simulink model "recoveryattempt_top_model"  (R2024b)
settings: Solver=VariableStepAuto  StartTime=0.0  StopTime=1000  FixedStep=0.001  RelTol=1e-6  EnableMultiTasking=on
undefined symbols (not defined in the file): ClassLabel, ClassValidity, controller, gray, imageEnums, images, pointsOfWay, vehicle, world, X, Y, Z
libraries: sm_lib x44, simulink x7, nesl_utility x7, slpidlib x2, deeplib x1, dspstat3 x1, robotmobilelib x1
(part 1 of 2)
settings Model: Creator=The MathWorks, Inc.  LastModifiedBy=carla
settings SolverCC: AlgebraicLoopSolver=TrustRegion  AutoInsertRateTranBlk=on
settings DataIOCC: LimitDataPoints=on  ReturnWorkspaceOutputs=off
settings OptimizationCC: LifeSpan=inf
settings DebuggingCC: AlgebraicLoopMsg=none  UnconnectedInputMsg=warning  UnconnectedOutputMsg=warning  UnconnectedLineMsg=warning  AllowSymbolicDim=off  SFUnexpectedBacktrackingDiag=warning  SFNoUnconditionalDefaultTransitionDiag=warning  SFExecutionAtInitializationDiag=none  ArithmeticOperatorsInVariantConditions=warning
settings ModelReferenceCC: EnableRefExpFcnMdlSchedulingChecks=on  PropagateSignalLabelsOutOfModel=off
settings SFSimCC: SimUseLocalCustomCode=off  CustomCodeUndefinedFunction=UseInterfaceOnly
settings RTWCC: RTWUseLocalCustomCode=off  GPUComputeCapability=3.5
settings CodeAppCC: StateflowObjectComments=on
settings GRTTargetCC: TargetLangStandard=C89/C90 (ANSI)
settings ConfigComp: CovMetricSettings=dw  CovSaveCumulativeToWorkspaceVar=on  CovSaveSingleToWorkspaceVar=on  CovExternalEMLEnable=off
settings ExplorerConfigSet: InternalSimMechanicsExplorerSettings="<ExplorerConfiguration><canonicalview>default</canonicalview><AnimationSetting><BasePlaybackSpeed>1.0</BasePlaybackSpeed><PlaybackSpeedFactor>4.0</PlaybackSpeedFactor></AnimationSetting><TilePanel><TileInfo><Tiles Columns=\"1\" Count=\"1\" Rows=\"1\"><Column Weight=\"1\"/><Row Weight=\"1\"/><Tile Height=\"1\" Width=\"1\" X=\"0\" Y=\"0\"/></Tiles></TileInfo><SceneInfo><SceneViewer><BGColor><R>0.60000002384185791</R><G>0.60000002384185791</G><B>0.60000002384185791</B></BGColor><Camera><DoPerspective>off</DoPerspective><Position><X>30.3692307922621794</X><Y>-2.86922998928845274</Y><Z>15.3692305721881048</Z></Position><Center><X>14.9999996252394148</X><Y>12.5000011777343119</Y><Z>-5.94834646427955249e-07</Z></Center><Up><X>-0.408248290463863073</X><Y>0.408248290463863073</Y><Z>0.816496580927726145</Z></Up><ViewLimDist>1</ViewLimDist><YLim>15.7961190654270691</YLim><XLim>27.3119994163513198</XLim></Camera></SceneViewer></SceneInfo></TilePanel><MechEditorPanel><Cameras/><GfxPanelCameraMap/><VideoCreator><PlaybackSpeedRatio>4.0</PlaybackSpeedRatio><FrameRate>30</FrameRate><VideoFormat>MPEG-4</VideoFormat><FrameSize>auto</FrameSize></VideoCreator></MechEditorPanel></ExplorerConfiguration>"

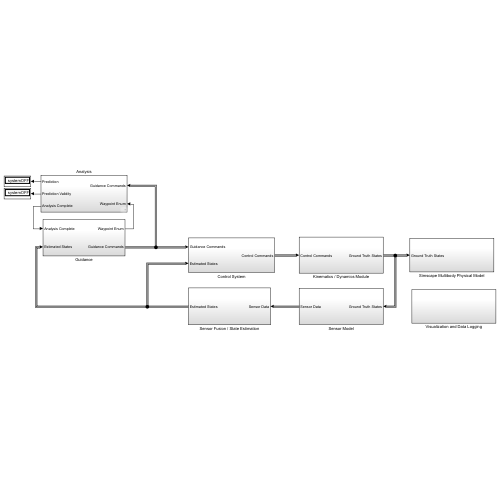
[thumbnail: Simulink's stored preview of the top-level diagram]
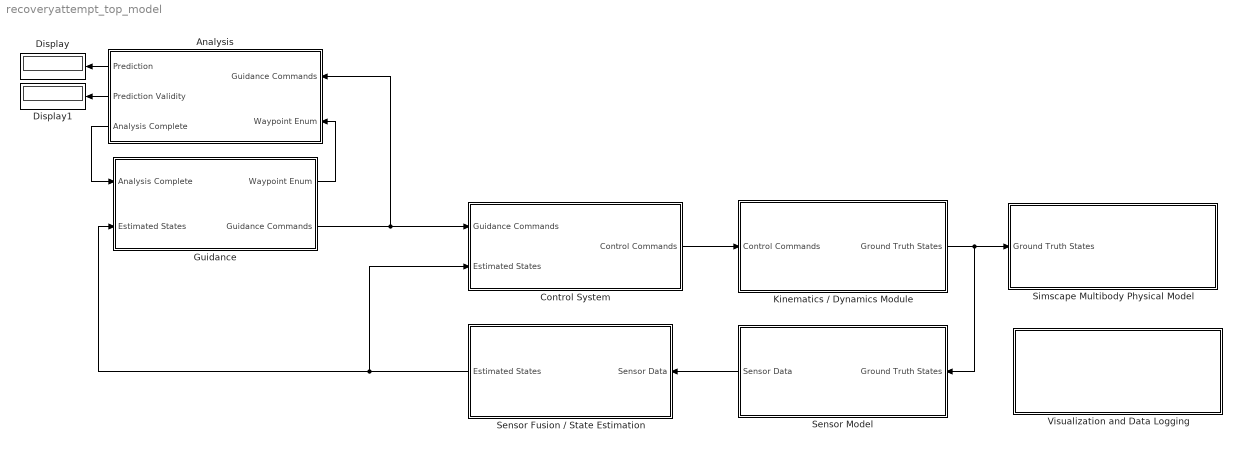
== system recoveryattempt_top_model ==
  Analysis : Subsystem
  Control System : Subsystem
  Display : Display
  Display1 : Display
  Guidance : Subsystem
  Kinematics / Dynamics Module : Subsystem
  Sensor Fusion / State Estimation : Subsystem
  Sensor Model : Subsystem
  Simscape Multibody Physical Model : Subsystem
  Visualization and Data Logging : Subsystem
  wires:
  Sensor Model/1(Sensor Data) -> Sensor Fusion / State Estimation/1(Sensor Data)
  Control System/1(Control Commands) -> Kinematics / Dynamics Module/1(Control Commands)
  Kinematics / Dynamics Module/1(Ground Truth States) -> Simscape Multibody Physical Model/1(Ground Truth States), Sensor Model/1(Ground Truth States)
  Sensor Fusion / State Estimation/1(Estimated States) -> Control System/2(Estimated States), Guidance/2(Estimated States)
  Analysis/1(Prediction) -> Display/1
  Guidance/2(Guidance Commands) -> Analysis/1(Guidance Commands), Control System/1(Guidance Commands)
  Analysis/3(Analysis Complete) -> Guidance/1(Analysis Complete)
  Guidance/1(Waypoint Enum) -> Analysis/2(Waypoint Enum)
  Analysis/2(Prediction Validity) -> Display1/1

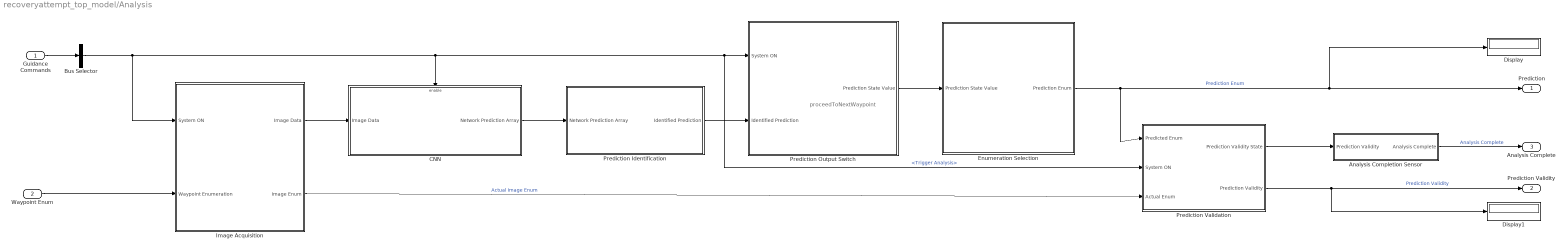
== system recoveryattempt_top_model/Analysis ==
  note: proceedToNextWaypoint
  Guidance Commands : Inport
  Waypoint Enum : Inport  Port=2
  Analysis Completion Sensor : Subsystem
  Bus Selector : BusSelector  OutputSignals=Process Commands.Trigger Analysis
  CNN : Subsystem
  Display : Display
  Display1 : Display
  Enumeration Selection : Subsystem
  Image Acquisition : Subsystem
  Prediction Identification : Subsystem
  Prediction Output Switch : Subsystem
  Prediction Validation : Subsystem
  Prediction : Outport
  Prediction Validity : Outport  Port=2
  Analysis Complete : Outport  Port=3
  wires:
  Waypoint Enum/1 -> Image Acquisition/2(Waypoint Enumeration)
  Image Acquisition/1(Image Data) -> CNN/1(Image Data)
  Bus Selector/1 -> Image Acquisition/1(System ON), CNN/Enable, Prediction Validation/2(System ON), Prediction Output Switch/1(System ON)  "<Trigger Analysis>"
  Guidance Commands/1 -> Bus Selector/1
  Prediction Identification/1(Identified Prediction) -> Prediction Output Switch/2(Identified Prediction)
  CNN/1(Network Prediction Array) -> Prediction Identification/1(Network Prediction Array)
  Enumeration Selection/1(Prediction Enum) -> Prediction Validation/1(Predicted Enum), Prediction/1, Display/1  "Prediction Enum"
  Prediction Output Switch/1(Prediction State Value) -> Enumeration Selection/1(Prediction State Value)
  Image Acquisition/2(Image Enum) -> Prediction Validation/3(Actual Enum)  "Actual Image Enum"
  Prediction Validation/2(Prediction Validity) -> Display1/1, Prediction Validity/1  "Prediction Validity"
  Analysis Completion Sensor/1(Analysis Complete) -> Analysis Complete/1  "Analysis Complete"
  Prediction Validation/1(Prediction Validity State) -> Analysis Completion Sensor/1(Prediction Validity)

== system recoveryattempt_top_model/Control System ==
  Guidance Commands : Inport
  Estimated States : Inport  Port=2
  Bus Selector : BusSelector  OutputSignals=Target Waypoints,Event Flags.Target Waypoint Reached
  Bus Selector1 : BusSelector  OutputSignals=True Position States
  Control Logic : Subsystem
  Control Commands : Outport
  wires:
  Estimated States/1 -> Bus Selector1/1
  Bus Selector/1 -> Control Logic/1(Target Waypoints)  "<Target Waypoints>"
  Guidance Commands/1 -> Bus Selector/1
  Control Logic/1(Control Commands) -> Control Commands/1
  Bus Selector1/1 -> Control Logic/3(Estimated Position)  "<True Position States>"
  Bus Selector/2 -> Control Logic/2(Target Waypoint Reached)  "<Target Waypoint Reached>"

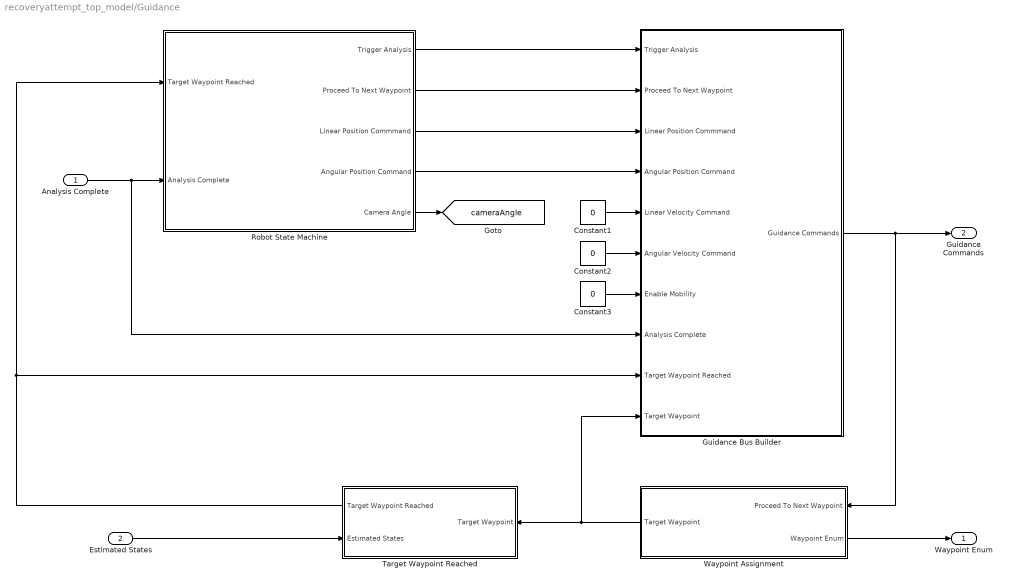
== system recoveryattempt_top_model/Guidance ==
  Analysis Complete : Inport
  Estimated States : Inport  Port=2
  Constant1 : Constant  Value=0
  Constant2 : Constant  Value=0
  Constant3 : Constant  Value=0
  Guidance Bus Builder : Subsystem
  Robot State Machine : Subsystem
  Target Waypoint Reached : Subsystem
      settings: PortSchema="{\"entries\":[{\"content\":{\"sides\":[{\"content\":{\"connectorIds\":[\"Out1\",\"In1\"]},\"type\":\"ConnectorPlacement.EquallySpacedRectSide\",\"uuid\":\"d7010085-5ef5-4f49-a809-03aff96e46a3\"},{\"content\":{\"connectorIds\":[\"In2\"],\"side\":\"RIGHT\"},\"type\":\"ConnectorPlacement.EquallySpacedRectSide\",\"uuid\":\"23b66111-6f3c-45e8-b3ba-0f5bee8484ca\"},{\"content\":{\"side\":\"TOP\"},\"type\":\"ConnectorPlacement.EquallySpacedRectSide\",\"uuid\":\"a521ae1c-357f-4992-b141-24939590eede\"}]},\"type\":\"ConnectorPlacement.EquallySpacedConnector\",\"uuid\":\"a962b4e6-4c12-48b9-996e-c7d697d970f0\"}],\"packageUris\":[\"http://schema.mathworks.com/mf0/Connector/R2020b\"],\"version\":\"1.0\"}"
  "Waypoint Assignment " : Subsystem
      settings: PortSchema="{\"entries\":[{\"content\":{\"sides\":[{\"content\":{\"connectorIds\":[\"In1\",\"Out2\"]},\"type\":\"ConnectorPlacement.EquallySpacedRectSide\",\"uuid\":\"23aedb4f-9300-4426-912f-0e2d5fd3b29f\"},{\"content\":{\"connectorIds\":[\"Out1\"],\"side\":\"RIGHT\"},\"type\":\"ConnectorPlacement.EquallySpacedRectSide\",\"uuid\":\"0851e076-2bde-4b70-9977-919ee7e7eb4f\"},{\"content\":{\"side\":\"TOP\"},\"type\":\"ConnectorPlacement.EquallySpacedRectSide\",\"uuid\":\"d0edf62d-75f3-4cec-8020-5fb7633b53e3\"}]},\"type\":\"ConnectorPlacement.EquallySpacedConnector\",\"uuid\":\"92e9c851-2c74-435e-8a22-f69b21df6f3e\"}],\"packageUris\":[\"http://schema.mathworks.com/mf0/Connector/R2020b\"],\"version\":\"1.0\"}"
  Waypoint Enum : Outport
  Guidance Commands : Outport  Port=2
  tag scope: cameraAngle=global
  wires:
  Robot State Machine/1(Trigger Analysis) -> Guidance Bus Builder/1(Trigger Analysis)
  Constant1/1 -> Guidance Bus Builder/5(Linear Velocity Command)
  Constant2/1 -> Guidance Bus Builder/6(Angular Velocity Command)
  Robot State Machine/4(Angular Position Command) -> Guidance Bus Builder/4(Angular Position Command)
  Robot State Machine/3(Linear Position Commmand) -> Guidance Bus Builder/3(Linear Position Commmand)
  Constant3/1 -> Guidance Bus Builder/7(Enable Mobility)
  Analysis Complete/1 -> Robot State Machine/2(Analysis Complete), Guidance Bus Builder/8(Analysis Complete)
  Robot State Machine/2(Proceed To Next Waypoint) -> Guidance Bus Builder/2(Proceed To Next Waypoint)
  Target Waypoint Reached/1(Target Waypoint Reached) -> Guidance Bus Builder/9(Target Waypoint Reached), Robot State Machine/1(Target Waypoint Reached)
  Guidance Bus Builder/1(Guidance Commands) -> Guidance Commands/1, "Waypoint Assignment "/1(Proceed To Next Waypoint)
  "Waypoint Assignment "/1(Target Waypoint) -> Guidance Bus Builder/10(Target Waypoint), Target Waypoint Reached/2(Target Waypoint)
  Estimated States/1 -> Target Waypoint Reached/1(Estimated States)
  Robot State Machine/5(Camera Angle) -> [cameraAngle]
  "Waypoint Assignment "/2(Waypoint Enum) -> Waypoint Enum/1

== system recoveryattempt_top_model/Kinematics // Dynamics Module ==
  Control Commands : Inport
  Bus Creator : BusCreator  Inputs=3
  Bus Creator1 : BusCreator  Inputs=3
  Bus Creator2 : BusCreator  Inputs=2
  Bus Selector : BusSelector  OutputSignals=Linear Velocity Command,Angular Velocity Command
  Demux1 : Demux  Outputs=3
  Demux2 : Demux  Outputs=3
  Differential Drive Kinematic Model : robotmobilelib/Differential Drive Kinematic Model  VehicleInputs=Vehicle Speed & Heading Angular Velocity  WheelRadius=vehicle.wheel.radius  WheelSpeedRange=[-inf inf]  TrackWidth=vehicle.wheel.width  InitialState=init.vehicle.state  SimulateUsing=Interpreted execution
  Ground Truth States : Outport
  wires:
  Bus Selector/1 -> Differential Drive Kinematic Model/1  "<Linear Velocity Command>"
  Bus Selector/2 -> Differential Drive Kinematic Model/2  "<Angular Velocity Command>"
  Control Commands/1 -> Bus Selector/1
  Differential Drive Kinematic Model/1 -> Demux1/1
  Demux1/2 -> Bus Creator/2  "True Position Y"
  Demux1/1 -> Bus Creator/1  "True Position X"
  Demux1/3 -> Bus Creator/3  "True Orientation"
  Differential Drive Kinematic Model/2 -> Demux2/1
  Demux2/1 -> Bus Creator1/1  "True Linear Velocity X"
  Demux2/3 -> Bus Creator1/3  "True Angular Velocity"
  Demux2/2 -> Bus Creator1/2  "True Linear Velocity Y"
  Bus Creator/1 -> Bus Creator2/1  "True Position States"
  Bus Creator1/1 -> Bus Creator2/2  "True Velocity States"
  Bus Creator2/1 -> Ground Truth States/1  "Ground Truth States"

== system recoveryattempt_top_model/Sensor Fusion // State Estimation ==
  Sensor Data : Inport
  Bus Creator : BusCreator  Inputs=2
  Bus Selector : BusSelector  OutputSignals=True Position States,True Velocity States
  Sensor Fusion : Subsystem
  Estimated States : Outport
  wires:
  Sensor Data/1 -> Bus Selector/1  "Sensor Data"
  Bus Creator/1 -> Estimated States/1  "Estimated States"
  Bus Selector/1 -> Sensor Fusion/1(In1)  "<True Position States>"
  Bus Selector/2 -> Sensor Fusion/2(In2)  "<True Velocity States>"
  Sensor Fusion/1(Out1) -> Bus Creator/1
  Sensor Fusion/2(Out2) -> Bus Creator/2

== system recoveryattempt_top_model/Sensor Model ==
  Ground Truth States : Inport
  Sensors : Subsystem
  Switch : simulink/Signal Routing/Manual Variant Source  NumChoices=2  LabelModeActiveChoice=V_1
  True Feedthrough : Subsystem
  Sensor Data : Outport
  wires:
  Switch/1 -> Sensor Data/1
  Ground Truth States/1 -> True Feedthrough/1(Ground Truth States), Sensors/1(Ground Truth States)
  Sensors/1(Simulated Raw Sensor Data) -> Switch/1  "Sensor Data"
  True Feedthrough/1(True Feedthrough Sensor Data) -> Switch/2  "Sensor Data"

== system recoveryattempt_top_model/Simscape Multibody Physical Model ==
  Ground Truth States : Inport
  Bus Creator : BusCreator  Inputs=1
  Bus Selector : BusSelector  OutputSignals=True Position States
  Bus Selector1 : BusSelector  OutputSignals=Camera Angle
  Simscape Model : Subsystem
  wires:
  Ground Truth States/1 -> Bus Selector/1
  Bus Selector/1 -> Simscape Model/1(True Position States)  "<True Position States>"
  Bus Selector1/1 -> Simscape Model/2(Peripheral Commands)  "<Camera Angle>"
  [cameraAngle] -> Bus Creator/1  "Camera Angle"
  Bus Creator/1 -> Bus Selector1/1  "Peripheral Commands"

== system recoveryattempt_top_model/Visualization and Data Logging ==

== system recoveryattempt_top_model/Analysis/Analysis Completion Sensor ==
  Prediction Validity : Inport
  Compare To Constant2 : simulink/Logic and Bit Operations/Compare To Constant  relop=<  const=2  OutDataTypeStr=boolean
  Display : Display
  Display1 : Display
  Analysis Complete : Outport
  wires:
  Prediction Validity/1 -> Display/1, Compare To Constant2/1
  Compare To Constant2/1 -> Analysis Complete/1, Display1/1

== system recoveryattempt_top_model/Analysis/CNN ==
  Image Data : Inport
  <Trigger Analysis> : EnablePort
  Predict : deeplib/Predict  Network=Network from MAT-file  NetworkFunction=squeezenet  NetworkFilePath=cleanTomatoNet.mat  MiniBatchSize=128  InputDataFormats={'',''}  Predictions=on  Activations={}  ForceInterpretedSim=off  EnableDLNetwork=on  LastKnownNetworkFilePath=''  LastKnownNetworkTimeStamp=''
  Network Prediction Array : Outport
  wires:
  Image Data/1 -> Predict/1
  Predict/1 -> Network Prediction Array/1

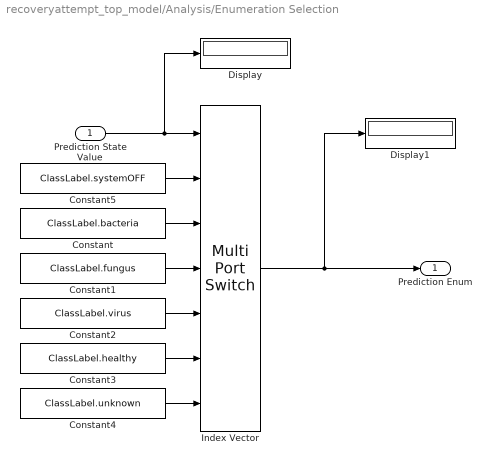
== system recoveryattempt_top_model/Analysis/Enumeration Selection ==
  Prediction State Value : Inport
  Constant : Constant  Value=ClassLabel.bacteria
  Constant1 : Constant  Value=ClassLabel.fungus
  Constant2 : Constant  Value=ClassLabel.virus
  Constant3 : Constant  Value=ClassLabel.healthy
  Constant4 : Constant  Value=ClassLabel.unknown
  Constant5 : Constant  Value=ClassLabel.systemOFF
  Display : Display
  Display1 : Display
  Index Vector : MultiPortSwitch  DataPortOrder=Zero-based contiguous  Inputs=6  zeroidx=on  SaturateOnIntegerOverflow=off  InputSameDT=off
  Prediction Enum : Outport
  wires:
  Index Vector/1 -> Prediction Enum/1, Display1/1
  Constant5/1 -> Index Vector/2
  Constant3/1 -> Index Vector/6
  Constant/1 -> Index Vector/3
  Constant4/1 -> Index Vector/7
  Constant1/1 -> Index Vector/4
  Constant2/1 -> Index Vector/5
  Prediction State Value/1 -> Index Vector/1, Display/1

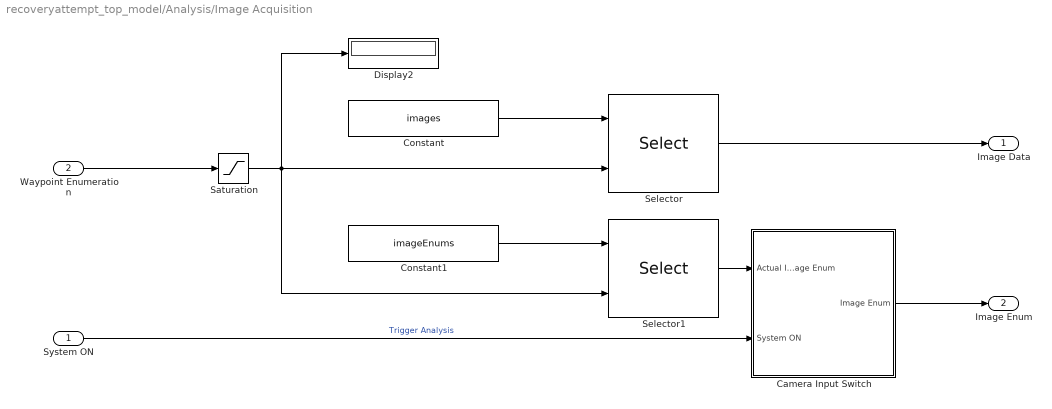
== system recoveryattempt_top_model/Analysis/Image Acquisition ==
  System ON : Inport
  Waypoint Enumeration : Inport  Port=2
  Camera Input Switch : Subsystem
  Constant : Constant  Value=images
  Constant1 : Constant  Value=imageEnums
  Display2 : Display
  Saturation : Saturate  UpperLimit=length(pointsOfWay)-1  LowerLimit=1
  Selector : Selector  NumberOfDimensions=4  InputPortWidth=3  IndexOptions=Select all,Select all,Select all,Index vector (port)  Indices=[1 3],1,1,1  OutputSizes=1,1,1,1
  Selector1 : Selector  InputPortWidth=36  IndexOptions=Index vector (port)  Indices=[1 3]  OutputSizes=1
  Image Data : Outport
  Image Enum : Outport  Port=2
  wires:
  Selector/1 -> Image Data/1
  Constant/1 -> Selector/1
  Constant1/1 -> Selector1/1
  Camera Input Switch/1(Image Enum) -> Image Enum/1
  Selector1/1 -> Camera Input Switch/1(Actual Image Enum)
  System ON/1 -> Camera Input Switch/2(System ON)  "Trigger Analysis"
  Waypoint Enumeration/1 -> Saturation/1
  Saturation/1 -> Selector1/2, Display2/1, Selector/2

== system recoveryattempt_top_model/Analysis/Prediction Identification ==
  Network Prediction Array : Inport
  Display : Display
  Display1 : Display
  Maximum : dspstat3/Maximum  operation=maximum  fcn=Index  indexBase=One  operateOver=Each row  Dimension=1  InputProcessing=Columns as channels (frame based)  reset=None  roiEnable=off  roiType=Rectangles  roiPortion=Entire ROI  roiOutput=Individual statistics for each ROI  roiFlag=off  roundingMode=Floor  overflowMode=off  accumDataTypeStr=Inherit: Same as product output  accumLastDataTypeStr=Inherit: Same as product output
  Identified Prediction : Outport
  wires:
  Network Prediction Array/1 -> Maximum/1, Display/1
  Maximum/1 -> Identified Prediction/1, Display1/1

== system recoveryattempt_top_model/Analysis/Prediction Output Switch ==
  System ON : Inport
  Identified Prediction : Inport  Port=2
  CNN OFF Value : Constant  Value=0
  Display : Display
  Display1 : Display
  Switch : Switch  Criteria=u2 > Threshold  SaturateOnIntegerOverflow=off  InputSameDT=off
  Prediction State Value : Outport
  wires:
  CNN OFF Value/1 -> Switch/3
  Switch/1 -> Prediction State Value/1, Display1/1
  Identified Prediction/1 -> Switch/1, Display/1
  System ON/1 -> Switch/2

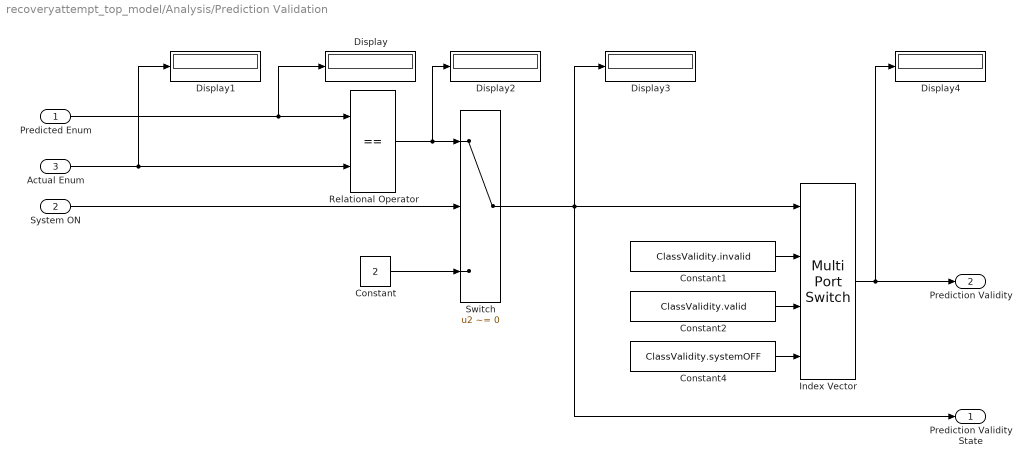
== system recoveryattempt_top_model/Analysis/Prediction Validation ==
  Predicted Enum : Inport
  System ON : Inport  Port=2
  Actual Enum : Inport  Port=3
  Constant : Constant  Value=2
  Constant1 : Constant  Value=ClassValidity.invalid
  Constant2 : Constant  Value=ClassValidity.valid
  Constant4 : Constant  Value=ClassValidity.systemOFF
  Display{,1..4} (5 alike) : Display
  Index Vector : MultiPortSwitch  DataPortOrder=Zero-based contiguous  zeroidx=on  SaturateOnIntegerOverflow=off  InputSameDT=off
  Relational Operator : RelationalOperator  Operator===  OutDataTypeStr=boolean  RndMeth=Simplest  InputSameDT=off
  Switch : Switch  Criteria=u2 ~= 0  SaturateOnIntegerOverflow=off  InputSameDT=off
  Prediction Validity State : Outport
  Prediction Validity : Outport  Port=2
  wires:
  Relational Operator/1 -> Display2/1, Switch/1
  Actual Enum/1 -> Relational Operator/2, Display1/1
  Switch/1 -> Display3/1, Prediction Validity State/1, Index Vector/1
  Constant/1 -> Switch/3
  Predicted Enum/1 -> Display/1, Relational Operator/1
  Constant1/1 -> Index Vector/2
  Constant2/1 -> Index Vector/3
  System ON/1 -> Switch/2
  Constant4/1 -> Index Vector/4
  Index Vector/1 -> Prediction Validity/1, Display4/1

== system recoveryattempt_top_model/Control System/Control Logic ==
  Target Waypoints : Inport
  Target Waypoint Reached : Inport  Port=2
  Estimated Position : Inport  Port=3
  Bearing Calculation : Subsystem
  Bus Selector : BusSelector  OutputSignals=True Position X,True Position Y,True Orientation
  PID Controllers : Subsystem
  Position Hold : Subsystem
  Possition Error Calculation : Subsystem
  Range Calculation : Subsystem
  Control Commands : Outport
  wires:
  Target Waypoints/1 -> Possition Error Calculation/3(Target Waypoints)
  Estimated Position/1 -> Bus Selector/1
  Bus Selector/3 -> PID Controllers/3(Robot Bearing)  "<True Orientation>"
  Position Hold/1(Control Commands) -> Control Commands/1
  Possition Error Calculation/1(Position Error) -> Range Calculation/1(Position Error), Bearing Calculation/1(Position Error)
  Bus Selector/1 -> Possition Error Calculation/1(Position X)  "<True Position X>"
  Bus Selector/2 -> Possition Error Calculation/2(Position Y)  "<True Position Y>"
  PID Controllers/1(PID Effort) -> Position Hold/2(PID Effort)
  Range Calculation/1(Target Range) -> PID Controllers/1(Range)
  Target Waypoint Reached/1 -> Position Hold/1(Target Waypoint Reached)
  Bearing Calculation/1(Target Bearing) -> PID Controllers/2(Final Target Bearing)

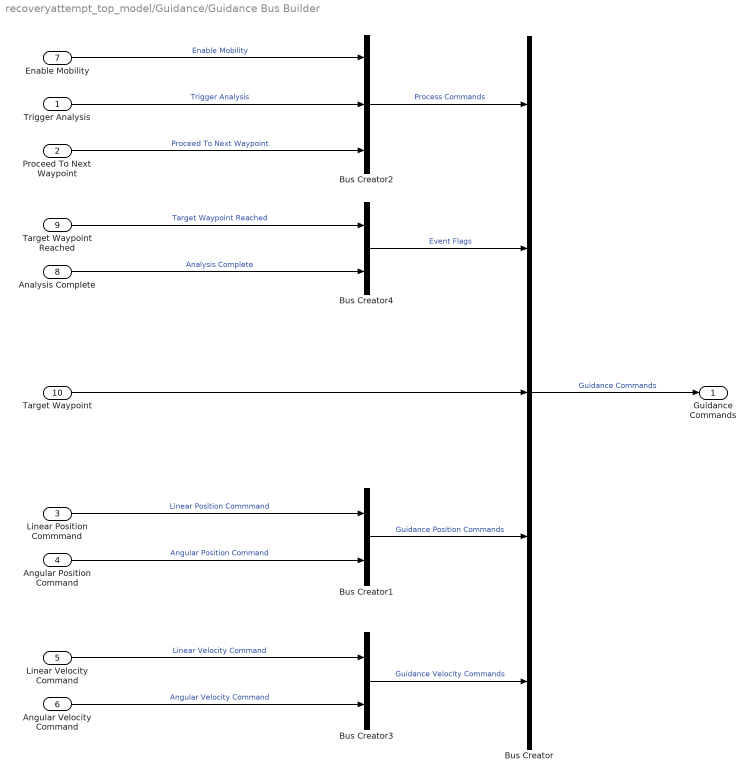
== system recoveryattempt_top_model/Guidance/Guidance Bus Builder ==
  Trigger Analysis : Inport
  Proceed To Next Waypoint : Inport  Port=2
  Linear Position Commmand : Inport  Port=3
  Angular Position Command : Inport  Port=4
  Linear Velocity Command : Inport  Port=5
  Angular Velocity Command : Inport  Port=6
  Enable Mobility : Inport  Port=7
  Analysis Complete : Inport  Port=8
  Target Waypoint Reached : Inport  Port=9
  Target Waypoint : Inport  Port=10
  Bus Creator : BusCreator  Inputs=5
  Bus Creator1 : BusCreator  Inputs=2
  Bus Creator2 : BusCreator  Inputs=3
  Bus Creator3 : BusCreator  Inputs=2
  Bus Creator4 : BusCreator  Inputs=2
  Guidance Commands : Outport
  wires:
  Angular Position Command/1 -> Bus Creator1/2  "Angular Position Command"
  Bus Creator3/1 -> Bus Creator/5  "Guidance Velocity Commands"
  Linear Velocity Command/1 -> Bus Creator3/1  "Linear Velocity Command"
  Bus Creator2/1 -> Bus Creator/1  "Process Commands"
  Bus Creator1/1 -> Bus Creator/4  "Guidance Position Commands"
  Bus Creator/1 -> Guidance Commands/1  "Guidance Commands"
  Linear Position Commmand/1 -> Bus Creator1/1  "Linear Position Commmand"
  Angular Velocity Command/1 -> Bus Creator3/2  "Angular Velocity Command"
  Trigger Analysis/1 -> Bus Creator2/2  "Trigger Analysis"
  Enable Mobility/1 -> Bus Creator2/1  "Enable Mobility"
  Bus Creator4/1 -> Bus Creator/2  "Event Flags"
  Target Waypoint Reached/1 -> Bus Creator4/1  "Target Waypoint Reached"
  Analysis Complete/1 -> Bus Creator4/2  "Analysis Complete"
  Proceed To Next Waypoint/1 -> Bus Creator2/3  "Proceed To Next Waypoint"
  Target Waypoint/1 -> Bus Creator/3

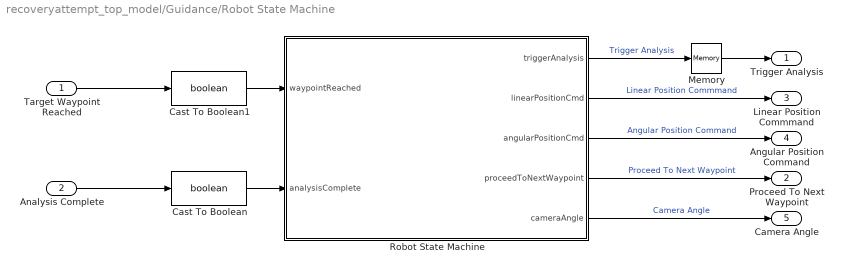
== system recoveryattempt_top_model/Guidance/Robot State Machine ==
  Target Waypoint Reached : Inport
  Analysis Complete : Inport  Port=2
  Cast To Boolean : DataTypeConversion  OutDataTypeStr=boolean  SaturateOnIntegerOverflow=off  RndMeth=Floor
  Cast To Boolean1 : DataTypeConversion  OutDataTypeStr=boolean  SaturateOnIntegerOverflow=off  RndMeth=Floor
  Memory : Memory
  Robot State Machine : Stateflow chart  TreatAsAtomicUnit=on
  Trigger Analysis : Outport
  Proceed To Next Waypoint : Outport  Port=2
  Linear Position Commmand : Outport  Port=3
  Angular Position Command : Outport  Port=4
  Camera Angle : Outport  Port=5
  wires:
  Target Waypoint Reached/1 -> Cast To Boolean1/1
  Analysis Complete/1 -> Cast To Boolean/1
  Robot State Machine/1(triggerAnalysis) -> Memory/1  "Trigger Analysis"
  Robot State Machine/2(linearPositionCmd) -> Linear Position Commmand/1  "Linear Position Commmand"
  Robot State Machine/3(angularPositionCmd) -> Angular Position Command/1  "Angular Position Command"
  Robot State Machine/4(proceedToNextWaypoint) -> Proceed To Next Waypoint/1  "Proceed To Next Waypoint"
  Cast To Boolean/1 -> Robot State Machine/2(analysisComplete)
  Cast To Boolean1/1 -> Robot State Machine/1(waypointReached)
  Robot State Machine/5(cameraAngle) -> Camera Angle/1  "Camera Angle"
  Memory/1 -> Trigger Analysis/1

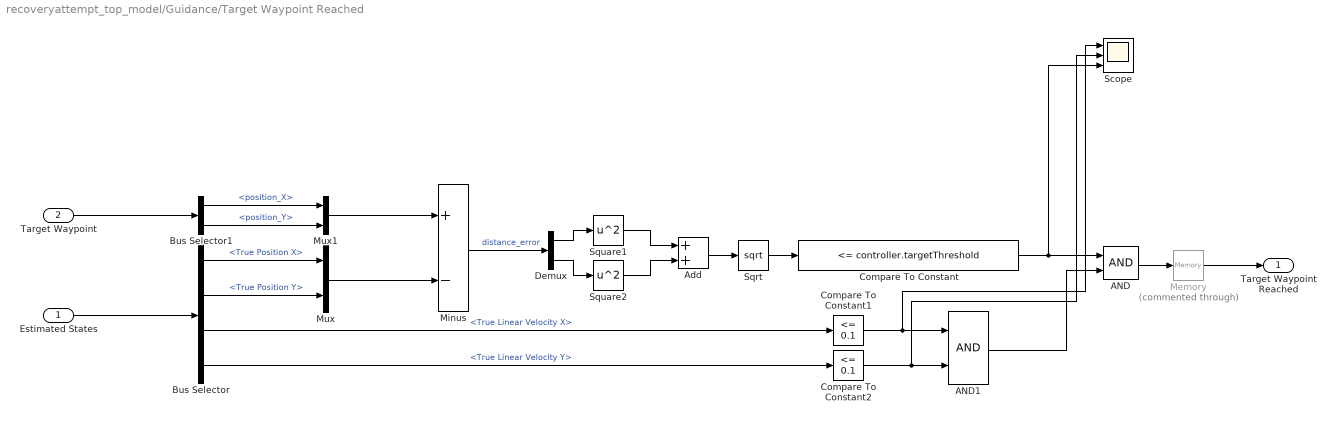
== system recoveryattempt_top_model/Guidance/Target Waypoint Reached ==
  Estimated States : Inport
  Target Waypoint : Inport  Port=2
  AND : Logic  AllPortsSameDT=off  OutDataTypeStr=boolean
  AND1 : Logic  AllPortsSameDT=off  OutDataTypeStr=boolean
  Add : Sum
  Bus Selector : BusSelector  OutputSignals=True Position States.True Position X,True Position States.True Position Y,True Velocity States.True Linear Velocity X,True Velocity States.True Linear Velocity Y
  Bus Selector1 : BusSelector  OutputSignals=position_X,position_Y
  Compare To Constant : simulink/Logic and Bit Operations/Compare To Constant  relop=<=  const=controller.targetThreshold  OutDataTypeStr=boolean
  Compare To Constant1 : simulink/Logic and Bit Operations/Compare To Constant  relop=<=  const=0.1  OutDataTypeStr=boolean
  Compare To Constant2 : simulink/Logic and Bit Operations/Compare To Constant  relop=<=  const=0.1  OutDataTypeStr=boolean
  Demux : Demux  Outputs=2
  Memory : Memory  Commented=through
  Minus : Sum  Inputs=+-
  Mux : Mux  Inputs=2
  Mux1 : Mux  Inputs=2
  Scope : Scope  NumInputPorts=3
  Sqrt : Sqrt
  Square1 : Math  Operator=square
  Square2 : Math  Operator=square
  Target Waypoint Reached : Outport
  wires:
  Bus Selector/1 -> Mux/1  "<True Position X>"
  Square1/1 -> Add/1
  Mux/1 -> Minus/2
  Bus Selector1/1 -> Mux1/1  "<position_X>"
  Sqrt/1 -> Compare To Constant/1
  Square2/1 -> Add/2
  Demux/2 -> Square2/1
  Mux1/1 -> Minus/1
  Demux/1 -> Square1/1
  Minus/1 -> Demux/1  "distance_error"
  Estimated States/1 -> Bus Selector/1
  Bus Selector/2 -> Mux/2  "<True Position Y>"
  Add/1 -> Sqrt/1
  Target Waypoint/1 -> Bus Selector1/1
  AND/1 -> Memory/1
  Memory/1 -> Target Waypoint Reached/1
  Compare To Constant/1 -> Scope/3, AND/1
  AND1/1 -> AND/2
  Compare To Constant1/1 -> Scope/1, AND1/1
  Compare To Constant2/1 -> Scope/2, AND1/2
  Bus Selector/3 -> Compare To Constant1/1  "<True Linear Velocity X>"
  Bus Selector/4 -> Compare To Constant2/1  "<True Linear Velocity Y>"
  Bus Selector1/2 -> Mux1/2  "<position_Y>"

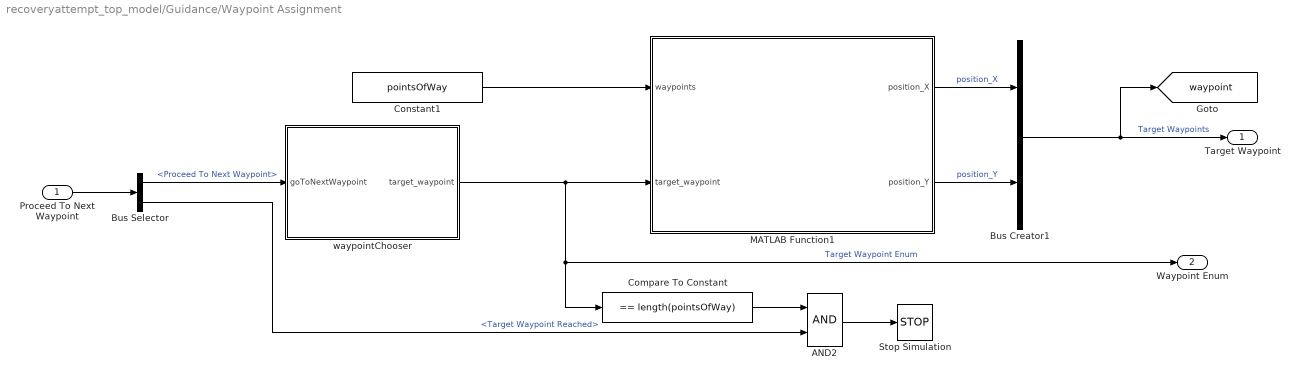
== system recoveryattempt_top_model/Guidance/Waypoint Assignment  ==
  Proceed To Next Waypoint : Inport
  AND2 : Logic  AllPortsSameDT=off  OutDataTypeStr=boolean
  Bus Creator1 : BusCreator  Inputs=2
  Bus Selector : BusSelector  OutputSignals=Process Commands.Proceed To Next Waypoint,Event Flags.Target Waypoint Reached
  Compare To Constant : simulink/Logic and Bit Operations/Compare To Constant  relop===  const=length(pointsOfWay)  OutDataTypeStr=boolean
  Constant1 : Constant  Value=pointsOfWay
  MATLAB Function1 : MATLAB Function  TreatAsAtomicUnit=on
  Stop Simulation : Stop
  waypointChooser : Subsystem
  Target Waypoint : Outport
  Waypoint Enum : Outport  Port=2
  tag scope: waypoint=global
  wires:
  Constant1/1 -> MATLAB Function1/1(waypoints)
  Bus Creator1/1 -> Target Waypoint/1, [waypoint]  "Target Waypoints"
  MATLAB Function1/2(position_Y) -> Bus Creator1/2  "position_Y"
  MATLAB Function1/1(position_X) -> Bus Creator1/1  "position_X"
  waypointChooser/1(target_waypoint) -> MATLAB Function1/2(target_waypoint), Compare To Constant/1, Waypoint Enum/1  "Target Waypoint Enum"
  Bus Selector/1 -> waypointChooser/1(goToNextWaypoint)  "<Proceed To Next Waypoint>"
  Proceed To Next Waypoint/1 -> Bus Selector/1
  Bus Selector/2 -> AND2/2  "<Target Waypoint Reached>"
  AND2/1 -> Stop Simulation/1
  Compare To Constant/1 -> AND2/1

== system recoveryattempt_top_model/Sensor Fusion // State Estimation/Sensor Fusion ==
  In1 : Inport
  In2 : Inport  Port=2
  Out1 : Outport
  Out2 : Outport  Port=2
  wires:
  In1/1 -> Out1/1
  In2/1 -> Out2/1

== system recoveryattempt_top_model/Sensor Model/Sensors ==
  Ground Truth States : Inport
  Bus Creator : BusCreator  Inputs=2
  Bus Selector : BusSelector  OutputSignals=True Position States,True Velocity States
  Camera : Subsystem
  Encoders : Subsystem  Commented=on
  GPS : Subsystem  Commented=on
  IMU : Subsystem  Commented=on
  LIDAR : Subsystem  Commented=on
  Simulated Raw Sensor Data : Outport
  wires:
  Ground Truth States/1 -> Bus Selector/1
  Bus Creator/1 -> Simulated Raw Sensor Data/1  "Simulated Raw Sensor Data"
  Camera/2(<True Position States>) -> Bus Creator/2
  Bus Selector/2 -> Camera/2(<True Velocity States - IN>)  "<True Velocity States>"
  Bus Selector/1 -> Camera/1(<True Position States - IN>)  "<True Position States>"
  Camera/1(<True Velocity States>) -> Bus Creator/1

== system recoveryattempt_top_model/Sensor Model/True Feedthrough ==
  Ground Truth States : Inport
  Bus Creator : BusCreator  Inputs=2
  Bus Selector : BusSelector  OutputSignals=True Position States,True Velocity States
  True Feedthrough Sensor Data : Outport
  wires:
  Bus Creator/1 -> True Feedthrough Sensor Data/1  "True Feedthrough Sensor Data"
  Ground Truth States/1 -> Bus Selector/1
  Bus Selector/1 -> Bus Creator/1  "<True Position States>"
  Bus Selector/2 -> Bus Creator/2  "<True Velocity States>"

== system recoveryattempt_top_model/Simscape Multibody Physical Model/Simscape Model ==
  True Position States : Inport
  Peripheral Commands : Inport  Port=2
  Target Indicator : Subsystem
  Vehicle Base : Subsystem
  World and Solver : Subsystem
  wires:
  True Position States/1 -> Vehicle Base/1(True Position States)
  Peripheral Commands/1 -> Vehicle Base/2(Peripheral Commands)
  connections:
  World and Solver/RConn1 -- Target Indicator/LConn1 -- Vehicle Base/LConn1

== system recoveryattempt_top_model/Analysis/Image Acquisition/Camera Input Switch ==
  Actual Image Enum : Inport
  System ON : Inport  Port=2
  CNN OFF Value : Constant  Value=ClassLabel.systemOFF
  Switch : Switch  Criteria=u2 > Threshold  SaturateOnIntegerOverflow=off  InputSameDT=off
  Image Enum : Outport
  wires:
  CNN OFF Value/1 -> Switch/3
  Switch/1 -> Image Enum/1
  Actual Image Enum/1 -> Switch/1
  System ON/1 -> Switch/2

== system recoveryattempt_top_model/Control System/Control Logic/Bearing Calculation ==
  Position Error : Inport
  Atan1 : Trigonometry  Operator=atan2
  Demux1 : Demux  Outputs=2
  Target Bearing : Outport
  wires:
  Demux1/2 -> Atan1/1
  Demux1/1 -> Atan1/2
  Atan1/1 -> Target Bearing/1
  Position Error/1 -> Demux1/1

== system recoveryattempt_top_model/Control System/Control Logic/PID Controllers ==
  Range : Inport
  Final Target Bearing : Inport  Port=2
  Robot Bearing : Inport  Port=3
  Angular Velocity Controller : slpidlib/PID Controller  Controller=PID  Form=Parallel  TimeDomain=Continuous-time  UseExternalTs=off  SampleTime=-1  IntegratorMethod=Forward Euler  FilterMethod=Forward Euler  ControllerParametersSource=internal  P=controller.angularVelocity.Kp  I=controller.angularVelocity.Ki  UseKiTs=off  D=controller.angularVelocity.Kd  UseExternalDerivativeSource=off  N=controller.angularVelocity.N  UseFilter=on  TunerSelectOption=Transfer Function Based (PID Tuner App)  InitialConditionSource=internal  InitialConditionForIntegrator=0  InitialConditionForFilter=0  DifferentiatorICPrevScaledInput=0  ExternalReset=none  TrackingMode=off  Kt=1  LimitOutput=off  SatLimitsSource=internal  UpperSaturationLimit=inf  LowerSaturationLimit=-inf  LinearizeAsGain=on  AntiWindupMode=none  Kb=1  LimitIntegrator=on  UpperIntegratorSaturationLimit=vehicle.maxAngularAcceleration  LowerIntegratorSaturationLimit=-vehicle.maxAngularAcceleration  POutMin=[]  POutMax=[]  IOutMin=[]  IOutMax=[]  DOutMin=[]  DOutMax=[]  NOutMin=[]  NOutMax=[]  SumOutMin=[]  SumOutMax=[]  SaturationOutMin=[]  SaturationOutMax=[]  PParamMin=[]  PParamMax=[]  IParamMin=[]  IParamMax=[]  DParamMin=[]  DParamMax=[]  NParamMin=[]  NParamMax=[]  KbParamMin=[]  KbParamMax=[]  KtParamMin=[]  KtParamMax=[]  KbOutMin=[]  KbOutMax=[]  KtOutMin=[]  KtOutMax=[]  IntegratorOutMin=[]  IntegratorOutMax=[]  FilterOutMin=[]  FilterOutMax=[]  SumI1OutMin=[]  SumI1OutMax=[]  SumI2OutMin=[]  SumI2OutMax=[]  SumI3OutMin=[]  SumI3OutMax=[]  SumI4OutMin=[]  SumI4OutMax=[]  SumDOutMin=[]  SumDOutMax=[]  DifferentiatorOutMin=[]  DifferentiatorOutMax=[]  FilterDiffOutCoefMin=[]  FilterDiffOutCoefMax=[]  ReciprocalOutMin=[]  ReciprocalOutMax=[]  SumDenOutMin=[]  SumDenOutMax=[]  SumNumOutMin=[]  SumNumOutMax=[]  DivideOutMin=[]  DivideOutMax=[]  UdiffTsProdOutMin=[]  UdiffTsProdOutMax=[]  NTsProdOutMin=[]  NTsProdOutMax=[]  UintegralTsProdOutMin=[]  UintegralTsProdOutMax=[]  UngainTsProdOutMin=[]  UngainTsProdOutMax=[]  ClampingZeroOutDataTypeStr=Inherit: Inherit via back propagation  ClampingZeroOutMin=[]  ClampingZeroOutMax=[]  FilterDenConstantOutDataTypeStr=Inherit: Inherit via back propagation  FilterDenConstantOutMin=[]  FilterDenConstantOutMax=[]  PCopyOutDataTypeStr=Inherit: Inherit via back propagation  PCopyOutMin=[]  PCopyOutMax=[]  NCopyOutDataTypeStr=Inherit: Inherit via back propagation  NCopyOutMin=[]  NCopyOutMax=[]  IntegratorContinuousStateAttributes=''  IntegratorStateMustResolveToSignalObject=off  IntegratorRTWStateStorageClass=Auto  FilterContinuousStateAttributes=''  FilterStateMustResolveToSignalObject=off  FilterRTWStateStorageClass=Auto  ParallelPVariant=InternalParameters  IdealPVariant=Disabled  IVariant=InternalParameters  DVariant=InternalParameters  IntegratorVariant=Continuous  SatVariant=Disabled  AWVariant=Passthrough  PCopyVariant=Disabled  TRVariant=Disabled  FdbkBlocksVariant=Forward  IdealPFdbkVariant=Disabled  SatFdbkVariant=Disabled  DerivativeFilterVariant=ContFilter  NVariant=InternalParameters  NCopyVariant=Disabled  FilterICVariant=InternalICsFilter  IntegratorICVariant=InternalICs  ExternalResetVariant=Disabled  TRSumVariant=Passthrough  SumFdbkVariant=Disabled  SumVariant=Sum_PID  TsampFilterVariant=InternalTs  TsampNgainVariant=Passthrough  TsampIntegralVariant=Disabled_SignalSpec  ExternalSaturationOutDataTypeStr=Inherit: Same as second input  DerivativeSourceVariant=ErrorSignal  PreIntVariant=InternalPreInt
  Linear Velocity Controller : slpidlib/PID Controller  Controller=PID  Form=Parallel  TimeDomain=Continuous-time  UseExternalTs=off  SampleTime=-1  IntegratorMethod=Forward Euler  FilterMethod=Forward Euler  ControllerParametersSource=internal  P=controller.linearVelocity.Kp  I=controller.linearVelocity.Ki  UseKiTs=off  D=controller.linearVelocity.Kd  UseExternalDerivativeSource=off  N=controller.linearVelocity.N  UseFilter=on  TunerSelectOption=Transfer Function Based (PID Tuner App)  InitialConditionSource=internal  InitialConditionForIntegrator=0  InitialConditionForFilter=0  DifferentiatorICPrevScaledInput=0  ExternalReset=none  TrackingMode=off  Kt=1  LimitOutput=off  SatLimitsSource=internal  UpperSaturationLimit=inf  LowerSaturationLimit=-inf  LinearizeAsGain=on  AntiWindupMode=none  Kb=1  LimitIntegrator=on  UpperIntegratorSaturationLimit=vehicle.maxLinearAcceleration  LowerIntegratorSaturationLimit=-vehicle.maxLinearAcceleration  POutMin=[]  POutMax=[]  IOutMin=[]  IOutMax=[]  DOutMin=[]  DOutMax=[]  NOutMin=[]  NOutMax=[]  SumOutMin=[]  SumOutMax=[]  SaturationOutMin=[]  SaturationOutMax=[]  PParamMin=[]  PParamMax=[]  IParamMin=[]  IParamMax=[]  DParamMin=[]  DParamMax=[]  NParamMin=[]  NParamMax=[]  KbParamMin=[]  KbParamMax=[]  KtParamMin=[]  KtParamMax=[]  KbOutMin=[]  KbOutMax=[]  KtOutMin=[]  KtOutMax=[]  IntegratorOutMin=[]  IntegratorOutMax=[]  FilterOutMin=[]  FilterOutMax=[]  SumI1OutMin=[]  SumI1OutMax=[]  SumI2OutMin=[]  SumI2OutMax=[]  SumI3OutMin=[]  SumI3OutMax=[]  SumI4OutMin=[]  SumI4OutMax=[]  SumDOutMin=[]  SumDOutMax=[]  DifferentiatorOutMin=[]  DifferentiatorOutMax=[]  FilterDiffOutCoefMin=[]  FilterDiffOutCoefMax=[]  ReciprocalOutMin=[]  ReciprocalOutMax=[]  SumDenOutMin=[]  SumDenOutMax=[]  SumNumOutMin=[]  SumNumOutMax=[]  DivideOutMin=[]  DivideOutMax=[]  UdiffTsProdOutMin=[]  UdiffTsProdOutMax=[]  NTsProdOutMin=[]  NTsProdOutMax=[]  UintegralTsProdOutMin=[]  UintegralTsProdOutMax=[]  UngainTsProdOutMin=[]  UngainTsProdOutMax=[]  ClampingZeroOutDataTypeStr=Inherit: Inherit via back propagation  ClampingZeroOutMin=[]  ClampingZeroOutMax=[]  FilterDenConstantOutDataTypeStr=Inherit: Inherit via back propagation  FilterDenConstantOutMin=[]  FilterDenConstantOutMax=[]  PCopyOutDataTypeStr=Inherit: Inherit via back propagation  PCopyOutMin=[]  PCopyOutMax=[]  NCopyOutDataTypeStr=Inherit: Inherit via back propagation  NCopyOutMin=[]  NCopyOutMax=[]  IntegratorContinuousStateAttributes=''  IntegratorStateMustResolveToSignalObject=off  IntegratorRTWStateStorageClass=Auto  FilterContinuousStateAttributes=''  FilterStateMustResolveToSignalObject=off  FilterRTWStateStorageClass=Auto  ParallelPVariant=InternalParameters  IdealPVariant=Disabled  IVariant=InternalParameters  DVariant=InternalParameters  IntegratorVariant=Continuous  SatVariant=Disabled  AWVariant=Passthrough  PCopyVariant=Disabled  TRVariant=Disabled  FdbkBlocksVariant=Forward  IdealPFdbkVariant=Disabled  SatFdbkVariant=Disabled  DerivativeFilterVariant=ContFilter  NVariant=InternalParameters  NCopyVariant=Disabled  FilterICVariant=InternalICsFilter  IntegratorICVariant=InternalICs  ExternalResetVariant=Disabled  TRSumVariant=Passthrough  SumFdbkVariant=Disabled  SumVariant=Sum_PID  TsampFilterVariant=InternalTs  TsampNgainVariant=Passthrough  TsampIntegralVariant=Disabled_SignalSpec  ExternalSaturationOutDataTypeStr=Inherit: Same as second input  DerivativeSourceVariant=ErrorSignal  PreIntVariant=InternalPreInt
  MATLAB Function : MATLAB Function  TreatAsAtomicUnit=on
  Minus4 : Sum  Inputs=+-
  Mux : Mux  Inputs=2
  Mux1 : Mux  Inputs=2
  Robot Heading Scope : Scope  NumInputPorts=2
  PID Effort : Outport
  wires:
  Linear Velocity Controller/1 -> Mux1/1
  Angular Velocity Controller/1 -> Mux1/2
  Minus4/1 -> MATLAB Function/1(heading_error)  "Heading Error"
  Range/1 -> Linear Velocity Controller/1
  Mux1/1 -> PID Effort/1
  Robot Bearing/1 -> Minus4/2, Mux/2
  MATLAB Function/1(heading_error_wrapped) -> Robot Heading Scope/2, Angular Velocity Controller/1
  Mux/1 -> Robot Heading Scope/1
  Final Target Bearing/1 -> Mux/1, Minus4/1

== system recoveryattempt_top_model/Control System/Control Logic/Position Hold ==
  Target Waypoint Reached : Inport
  PID Effort : Inport  Port=2
  Bus Creator : BusCreator  Inputs=2
  Constant : Constant  Value=[0 0]
  Demux : Demux  Outputs=2
  Rate Limiter : RateLimiter  RisingSlewLimit=vehicle.maxAngularAcceleration  FallingSlewLimit=-vehicle.maxAngularAcceleration  SampleTimeMode=inherited
  Rate Limiter1 : RateLimiter  RisingSlewLimit=vehicle.maxLinearAcceleration  FallingSlewLimit=-vehicle.maxLinearAcceleration  SampleTimeMode=inherited
  Saturation : Saturate  UpperLimit=vehicle.maxAngularVelocity  LowerLimit=-vehicle.maxAngularVelocity
  Saturation1 : Saturate  UpperLimit=vehicle.maxLinearVelocity  LowerLimit=-vehicle.maxLinearVelocity
  Switch : Switch  Criteria=u2 > Threshold  SaturateOnIntegerOverflow=off  InputSameDT=off
  Control Commands : Outport
  wires:
  PID Effort/1 -> Switch/3
  Rate Limiter1/1 -> Bus Creator/1  "Linear Velocity Command"
  Rate Limiter/1 -> Bus Creator/2  "Angular Velocity Command"
  Bus Creator/1 -> Control Commands/1  "Control Commands"
  Saturation/1 -> Rate Limiter/1
  Saturation1/1 -> Rate Limiter1/1
  Demux/1 -> Saturation1/1
  Demux/2 -> Saturation/1
  Switch/1 -> Demux/1
  Target Waypoint Reached/1 -> Switch/2
  Constant/1 -> Switch/1

== system recoveryattempt_top_model/Control System/Control Logic/Possition Error Calculation ==
  Position X : Inport
  Position Y : Inport  Port=2
  Target Waypoints : Inport  Port=3
  Minus3 : Sum  Inputs=+-
  Mux : Mux  Inputs=2
  Position Error : Outport
  wires:
  Mux/1 -> Minus3/2
  Position Y/1 -> Mux/2
  Target Waypoints/1 -> Minus3/1
  Minus3/1 -> Position Error/1
  Position X/1 -> Mux/1

== system recoveryattempt_top_model/Control System/Control Logic/Range Calculation ==
  Position Error : Inport
  Square Root1 : Sqrt
  Square2 : Math  Operator=square
  Sum of Elements : Sum  Inputs=+
  Target Range : Outport
  wires:
  Sum of Elements/1 -> Square Root1/1
  Square2/1 -> Sum of Elements/1
  Square Root1/1 -> Target Range/1  "Range"
  Position Error/1 -> Square2/1

== system recoveryattempt_top_model/Guidance/Waypoint Assignment /waypointChooser ==
  goToNextWaypoint : Inport
  Memory : Memory  InitialCondition=1  LinearizeMemory=on
  Saturation : Saturate  UpperLimit=length(pointsOfWay)  LowerLimit=1
  Triggered Subsystem : Subsystem  TreatAsAtomicUnit=on
  target_waypoint : Outport
  wires:
  Triggered Subsystem/1(target_waypoint) -> Saturation/1
  Saturation/1 -> Memory/1
  goToNextWaypoint/1 -> Triggered Subsystem/Trigger
  Memory/1 -> target_waypoint/1

== system recoveryattempt_top_model/Sensor Model/Sensors/Camera ==
  <True Position States - IN> : Inport
  <True Velocity States - IN> : Inport  Port=2
  MATLAB Function : MATLAB Function  TreatAsAtomicUnit=on
  Video Viewer : VideoViewer  Commented=on  colormapValue=gray(256)  FigPos=[2458 385 418 304]
  <True Velocity States> : Outport
  <True Position States> : Outport  Port=2
  wires:
  <True Position States - IN>/1 -> <True Position States>/1, MATLAB Function/1(pose)
  <True Velocity States - IN>/1 -> <True Velocity States>/1
  MATLAB Function/1(I) -> Video Viewer/1

== system recoveryattempt_top_model/Sensor Model/Sensors/Encoders ==
  In1 : Inport
  Out1 : Outport
  wires:
  In1/1 -> Out1/1

== system recoveryattempt_top_model/Sensor Model/Sensors/GPS ==
  In1 : Inport
  Out1 : Outport
  wires:
  In1/1 -> Out1/1

== system recoveryattempt_top_model/Sensor Model/Sensors/IMU ==
  In1 : Inport
  Out1 : Outport
  wires:
  In1/1 -> Out1/1

== system recoveryattempt_top_model/Sensor Model/Sensors/LIDAR ==
  In1 : Inport
  Out1 : Outport
  wires:
  In1/1 -> Out1/1

== system recoveryattempt_top_model/Simscape Multibody Physical Model/Simscape Model/Target Indicator ==
  Demux : Demux  Outputs=2
  Rectangular Joint : sm_lib/Joints/Rectangular Joint  JointMode=Normal  CompositeWrenchDir=FollowerOnBase  CompositeWrenchFrame=BaseFrame  SenseConstraintForce=off  SenseConstraintTorque=off  SenseTotalForce=off  SenseTotalTorque=off  PxPositionTargetSpecify=off  PxPositionTargetPriority=High  PxPositionTargetValue=0  PxPositionTargetValueUnits=m  PxVelocityTargetSpecify=off  PxVelocityTargetPriority=High  PxVelocityTargetValue=0  PxVelocityTargetValueUnits=m/s  PxEquilibriumPosition=0  PxEquilibriumPositionUnits=m  PxSpringStiffness=0  PxSpringStiffnessUnits=N/m  PxDampingCoefficient=0  PxDampingCoefficientUnits=N/(m/s)  PxLowerLimitSpecify=off  PxLowerLimitBound=-1  PxLowerLimitBoundUnits=m  PxLowerLimitStiffness=1e6  PxLowerLimitStiffnessUnits=N/m  PxLowerLimitDamping=1e3  PxLowerLimitDampingUnits=N/(m/s)  PxLowerLimitTransitionRegionWidth=1e-4  PxLowerLimitTransitionRegionWidthUnits=m  PxUpperLimitSpecify=off  PxUpperLimitBound=1  PxUpperLimitBoundUnits=m  PxUpperLimitStiffness=1e6  PxUpperLimitStiffnessUnits=N/m  PxUpperLimitDamping=1e3  PxUpperLimitDampingUnits=N/(m/s)  PxUpperLimitTransitionRegionWidth=1e-4  PxUpperLimitTransitionRegionWidthUnits=m  PxTorqueActuationMode=ComputedTorque  PxMotionActuationMode=InputMotion  PxSensePosition=off  PxSenseVelocity=off  PxSenseAcceleration=off  PxSenseTorqueForce=off  PxSenseLowerLimitTorqueForce=off  PxSenseUpperLimitTorqueForce=off  PyPositionTargetSpecify=off  PyPositionTargetPriority=High  PyPositionTargetValue=0  PyPositionTargetValueUnits=m  PyVelocityTargetSpecify=off  PyVelocityTargetPriority=High  PyVelocityTargetValue=0  PyVelocityTargetValueUnits=m/s  PyEquilibriumPosition=0  PyEquilibriumPositionUnits=m  PySpringStiffness=0  PySpringStiffnessUnits=N/m  PyDampingCoefficient=0  PyDampingCoefficientUnits=N/(m/s)  PyLowerLimitSpecify=off  PyLowerLimitBound=-1  PyLowerLimitBoundUnits=m  PyLowerLimitStiffness=1e6  PyLowerLimitStiffnessUnits=N/m  PyLowerLimitDamping=1e3  PyLowerLimitDampingUnits=N/(m/s)  PyLowerLimitTransitionRegionWidth=1e-4  PyLowerLimitTransitionRegionWidthUnits=m  PyUpperLimitSpecify=off  PyUpperLimitBound=1  PyUpperLimitBoundUnits=m  PyUpperLimitStiffness=1e6  PyUpperLimitStiffnessUnits=N/m  PyUpperLimitDamping=1e3  PyUpperLimitDampingUnits=N/(m/s)  PyUpperLimitTransitionRegionWidth=1e-4  PyUpperLimitTransitionRegionWidthUnits=m  PyTorqueActuationMode=ComputedTorque  PyMotionActuationMode=InputMotion  PySensePosition=off  PySenseVelocity=off  PySenseAcceleration=off  PySenseTorqueForce=off  PySenseLowerLimitTorqueForce=off  PySenseUpperLimitTorqueForce=off
  Simulink-PS Converter3 : nesl_utility/Simulink-PS Converter  PhysicalDomain=network_engine_domain  SubClassName=ps_input  LeftPortType=input  RightPortType=output  PseudoPeriodic=off  Frequencies=[]  NoiseDistribution=none  NoiseParameters=[]  Unit=1  AffineConversion=off  FilteringAndDerivatives=filter  SimscapeFilterOrder=2  InputFilterTimeConstant=0.001  UdotUserProvided=0
  Simulink-PS Converter4 : nesl_utility/Simulink-PS Converter  PhysicalDomain=network_engine_domain  SubClassName=ps_input  LeftPortType=input  RightPortType=output  PseudoPeriodic=off  Frequencies=[]  NoiseDistribution=none  NoiseParameters=[]  Unit=1  AffineConversion=off  FilteringAndDerivatives=filter  SimscapeFilterOrder=2  InputFilterTimeConstant=0.001  UdotUserProvided=0
  Spherical Solid : sm_lib/Body Elements/Spherical Solid  SphereRadius=target.radius  SphereRadiusUnits=m  ExportEntireGeometry=off  InertiaType=CalculateFromGeometry  BasedOnType=Mass  Density=1000  DensityUnits=kg/m^3  Mass=0  MassUnits=kg  CenterOfMass=[0 0 0]  CenterOfMassUnits=m  MomentsOfInertia=[1 1 1]  MomentsOfInertiaUnits=kg*m^2  ProductsOfInertia=[0 0 0]  ProductsOfInertiaUnits=kg*m^2  GraphicType=FromGeometry  MarkerShape=Sphere  MarkerSize=10  GraphicVisPropType=SimpleVisualProperties  GraphicDiffuseColor=target.colour  GraphicOpacity=target.opacity  GraphicSpecularColor=[0.5 0.5 0.5 1.0]  GraphicAmbientColor=[0.15 0.15 0.15 1.0]  GraphicEmissiveColor=[0.0 0.0 0.0 1.0]  GraphicShininess=75  DoExposeReferenceFrame=on  SerializedFrames=<Frames/>
  Conn1 : PMIOPort  Side=Left
  wires:
  Demux/2 -> Simulink-PS Converter4/1
  Demux/1 -> Simulink-PS Converter3/1
  [waypoint] -> Demux/1
  connections:
  Simulink-PS Converter4/RConn1 -- Rectangular Joint/LConn3
  Rectangular Joint/RConn1 -- Spherical Solid/RConn1
  Simulink-PS Converter3/RConn1 -- Rectangular Joint/LConn2
  Rectangular Joint/LConn1 -- Conn1/RConn1

== system recoveryattempt_top_model/Simscape Multibody Physical Model/Simscape Model/Vehicle Base ==
  True Position States : Inport
  Peripheral Commands : Inport  Port=2
  Camera System : Subsystem
      settings: PortSchema="{\"entries\":[{\"content\":{\"sides\":[{\"content\":{\"connectorIds\":[\"LConn1\",\"In1\"]},\"type\":\"ConnectorPlacement.EquallySpacedRectSide\",\"uuid\":\"8fffb0c1-8e08-42dc-a89e-0bb2b361ba06\"},{\"content\":{\"side\":\"RIGHT\"},\"type\":\"ConnectorPlacement.EquallySpacedRectSide\",\"uuid\":\"e1761592-c124-42d7-8589-f246c81df988\"},{\"content\":{\"side\":\"TOP\"},\"type\":\"ConnectorPlacement.EquallySpacedRectSide\",\"uuid\":\"26792343-9fc4-426e-9919-a165cea725a9\"}]},\"type\":\"ConnectorPlacement.EquallySpacedConnector\",\"uuid\":\"2aa2b44c-9393-46bf-9a47-8db95130564c\"}],\"packageUris\":[\"http://schema.mathworks.com/mf0/Connector/R2020b\"],\"version\":\"1.0\"}"
  Front Left Wheel : Subsystem
  Front Right Wheel : Subsystem
  Rear Left Wheel1 : Subsystem
  Rear Right Wheel : Subsystem
  Subsystem : Subsystem
      settings: PortSchema="{\"entries\":[{\"content\":{\"sides\":[{\"content\":{\"connectorIds\":[\"LConn1\",\"In1\"]},\"type\":\"ConnectorPlacement.EquallySpacedRectSide\",\"uuid\":\"2a8e2290-7b0b-4ad0-b9c1-b7ab3e96c0f7\"},{\"content\":{\"connectorIds\":[\"RConn1\"],\"side\":\"RIGHT\"},\"type\":\"ConnectorPlacement.EquallySpacedRectSide\",\"uuid\":\"96b0eaee-bfd3-4351-bfb0-254a02911695\"},{\"content\":{\"side\":\"TOP\"},\"type\":\"ConnectorPlacement.EquallySpacedRectSide\",\"uuid\":\"b94364d8-c666-46cf-b6f3-d9ca1f8b044c\"}]},\"type\":\"ConnectorPlacement.EquallySpacedConnector\",\"uuid\":\"8821356c-4de8-4ea9-9249-6efa68ffc4bd\"}],\"packageUris\":[\"http://schema.mathworks.com/mf0/Connector/R2020b\"],\"version\":\"1.0\"}"
  Vehicle Base Chasis : Subsystem
      settings: PortSchema="{\"entries\":[{\"content\":{\"sides\":[{\"content\":{\"connectorIds\":[\"LConn1\",\"LConn2\"]},\"type\":\"ConnectorPlacement.EquallySpacedRectSide\",\"uuid\":\"09fe3aa5-c152-4c64-af2d-e4e22fceafa2\"},{\"content\":{\"connectorIds\":[\"RConn1\",\"RConn2\"],\"side\":\"RIGHT\"},\"type\":\"ConnectorPlacement.EquallySpacedRectSide\",\"uuid\":\"de7b1764-853d-48eb-939b-d4ad209edc2c\"},{\"content\":{\"side\":\"TOP\"},\"type\":\"ConnectorPlacement.EquallySpacedRectSide\",\"uuid\":\"49692483-3898-4392-9bcb-63fcf6451996\"},{\"content\":{\"connectorIds\":[\"RConn3\",\"RConn4\"],\"side\":\"BOTTOM\"},\"type\":\"ConnectorPlacement.EquallySpacedRectSide\",\"uuid\":\"37031ed8-38e9-47db-aede-addae70fadc1\"}]},\"type\":\"ConnectorPlacement.EquallySpacedConnector\",\"uuid\":\"6b211a4b-62db-4963-aba1-c087ec495b2b\"}],\"packageUris\":[\"http://schema.mathworks.com/mf0/Connector/R2020b\"],\"version\":\"1.0\"}"
  World Link : PMIOPort  Side=Left
  wires:
  True Position States/1 -> Subsystem/1(True Position States)
  Peripheral Commands/1 -> Camera System/1(Camera Angle)
  connections:
  Subsystem/LConn1 -- World Link/RConn1
  Vehicle Base Chasis/LConn1 -- Front Left Wheel/LConn1
  Rear Left Wheel1/LConn1 -- Vehicle Base Chasis/LConn2
  Vehicle Base Chasis/RConn3 -- Subsystem/RConn1
  Rear Right Wheel/LConn1 -- Vehicle Base Chasis/RConn2
  Front Right Wheel/LConn1 -- Vehicle Base Chasis/RConn1
  Camera System/LConn1 -- Vehicle Base Chasis/RConn4
